simulink model "MPC_1_QuadrotorModel"  (R2023b)
settings: Solver=VariableStepAuto  StartTime=0.0  StopTime=60  FixedStep=0.0005  MaxStep=0.05  RelTol=1e-3
InitFcn:
  | nlobj = init_nmpc();
values from neighbouring files (symbols this model uses):
  A_flap = [c_a, c_b, 0 ... (first row only)    [LQR_calculate.m]    (also in LQR_feedback.m; LQR_linearized_test.m; MPC_test.m; MPC_test_1.m)
  A_ind = [c_d, 0, 0 ... (first row only)    [LQR_calculate.m]    (also in LQR_feedback.m; LQR_linearized_test.m; MPC_test.m; MPC_test_1.m)
  C_drag = 0    [LQR_calculate.m]    (also in LQR_feedback.m = C_drag_arr(i); LQR_linearized_test.m = C_drag_arr(i); MPC_test.m = C_drag_arr(i); MPC_test_1.m = C_drag_arr(i))
  demp = 0    [LQR_feedback.m]    (also in LQR_linearized_test.m; MPC_params.m; MPC_test_1.m; initQuadrotorData.m)
  forward_1 = 20    [LQR_feedback.m]    (also in LQR_linearized_test.m; MPC_test_1.m)
  forward_2 = 20    [LQR_feedback.m]    (also in LQR_linearized_test.m; MPC_test_1.m)
  g = 9.81    [LQR_calculate.m]    (also in LQR_feedback.m = 9.8; LQR_linearized_test.m = 9.8; LQR_testing_gpt.m; MPC_params.m = 9.8)
  Ix = m/3*a^2/12+2*0.045*l^2    (= 0.00211347222222)    [LQR_calculate.m]    (also in LQR_feedback.m; LQR_linearized_test.m; LQR_testing_gpt.m = 0.0081; MPC_params.m)
  Iy = m/3*a^2/12+4*0.045*l^2    (= 0.00413847222222)    [LQR_calculate.m]    (also in LQR_feedback.m = 0.00211347222222; LQR_linearized_test.m = 0.00211347222222; LQR_testing_gpt.m = 0.0081; MPC_params.m = 0.00211347222222)
  Iz = m/3*a^2/4+2*0.045*l^2    (= 0.00229041666667)    [LQR_calculate.m]    (also in LQR_feedback.m = 0.00431541666667; LQR_linearized_test.m = 0.00431541666667; LQR_testing_gpt.m = 0.0142; MPC_params.m = 0.00431541666667)
  J = 2.5*10^(-6)    (= 2.5e-06)    [LQR_calculate.m]    (also in LQR_feedback.m; LQR_linearized_test.m; MPC_params.m; MPC_test.m)
  Ke = ke    (= 0.0073)    [LQR_calculate.m]    (also in LQR_feedback.m = 0.00734; LQR_linearized_test.m = 0.00734; MPC_params.m = 0.00734; MPC_test.m)
  kf = ks*r^2*airDensity*Sblade/2    (= 1.57565625e-05)    [LQR_calculate.m]    (also in LQR_feedback.m; LQR_linearized_test.m; MPC_params.m; MPC_test.m)
  Km = kt    (= 0.0073)    [LQR_calculate.m]    (also in LQR_feedback.m = 0.00734; LQR_linearized_test.m = 0.00734; MPC_params.m = 0.00734; MPC_test.m)
  kv = 1300    [LQR_feedback.m]    (also in LQR_linearized_test.m; MPC_test_1.m; initQuadrotorData.m)
  L = La    (= 5e-05)    [LQR_calculate.m]    (also in LQR_feedback.m = 0.0001; LQR_linearized_test.m = 0.0001; MPC_params.m = 0.0001; MPC_test.m)
  l = 0.15    [LQR_calculate.m]    (also in LQR_feedback.m; LQR_linearized_test.m; MPC_params.m; MPC_test.m)
  m = size(B, 2)    [LQR_calculate.m]    (also in LQR_feedback.m = 0.65; LQR_linearized_test.m = 0.65; LQR_testing_gpt.m = 1; MPC_params.m = 0.65)
  maxU = 16    [LQR_calculate.m]    (also in LQR_feedback.m; LQR_linearized_test.m; MPC_params.m; MPC_test.m = 11)
  Mode = 3    [LQR_feedback.m]    (also in LQR_linearized_test.m; MPC_test_1.m = 1)
  N = params.N    [MPC_test_1.m]    (also in initQuadrotorData.m)
  phi0 = 0    [LQR_feedback.m]    (also in LQR_linearized_test.m; MPC_test_1.m)
  psi0 = pi/2    (= 1.57079632679)    [LQR_feedback.m]    (also in LQR_linearized_test.m; MPC_test_1.m = 0)
  Qc = diag([500, 500, 500, 1, 1, 1, 1, 1, 10, 1, 1, 1])    [MPC_test_1.m]
  R = eye(4)    [LQR_calculate.m]    (also in LQR_feedback.m = 0.058; LQR_linearized_test.m = 0.058; LQR_testing_gpt.m = diag([0.1, 10, 100, 10]); MPC_params.m = 0.058)
  Rc = diag([1, 1, 1, 1])    [LQR_feedback.m]    (also in LQR_linearized_test.m; MPC_test_1.m = diag([0.1, 0.1, 0.1, 0.1]))
  rho = 1.225    [LQR_calculate.m]    (also in LQR_feedback.m; LQR_linearized_test.m; MPC_params.m; MPC_test.m)
  S = l*c*4+a*b    (= 0.0169)    [LQR_calculate.m]    (also in LQR_feedback.m; LQR_linearized_test.m; MPC_params.m; MPC_test.m)
  theta0 = 0    [LQR_feedback.m]    (also in LQR_linearized_test.m; MPC_test_1.m)
  total_time = 60    [LQR_feedback.m]    (also in LQR_linearized_test.m; MPC_test_1.m)
  U_ref = repmat(u_nominal', params.N, 1)    [MPC_test_1.m]    (also in initQuadrotorData.m)
  up_down = 5    [LQR_feedback.m]    (also in LQR_linearized_test.m; MPC_test_1.m)
  x0 = 0    [LQR_feedback.m]    (also in LQR_linearized_test.m; MPC_test_1.m; init_nmpc.m = zeros(nx,1))
  y0 = 0    [LQR_feedback.m]    (also in LQR_linearized_test.m; MPC_test_1.m)
  z0 = 0    [LQR_feedback.m]    (also in LQR_linearized_test.m; MPC_test_1.m)
libraries: mpclib x1, sharedtransform x1
settings Model: Creator=Degra  LastModifiedBy=Degra

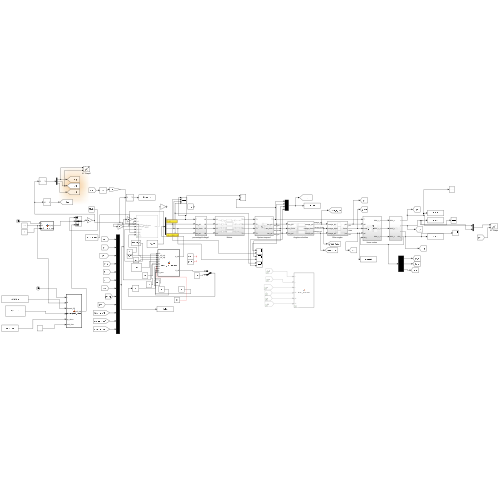
[thumbnail: Simulink's stored preview of the top-level diagram]
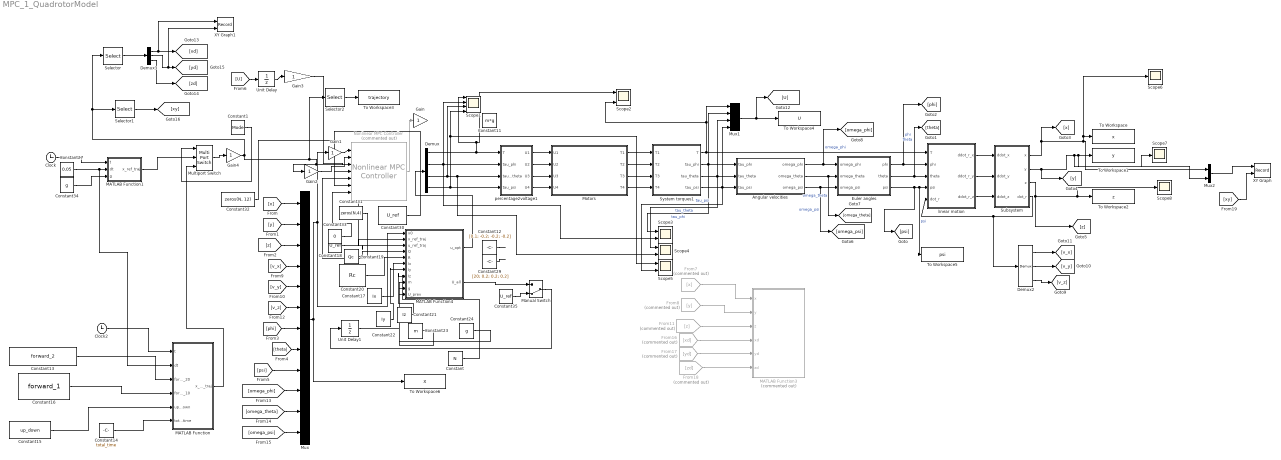
== system MPC_1_QuadrotorModel ==
  Angular velocities : Subsystem
  Clock : Clock
  Clock2 : Clock
  Constant : Constant  Value=N
  Constant1 : Constant  Value=Mode
  Constant11 : Constant  Value=m*g
  Constant12 : Constant  Value=[0.1; -0.2; -0.2; -0.2]
  Constant13 : Constant  Value=forward_2
  Constant14 : Constant  Value=total_time
  Constant15 : Constant  Value=up_down
  Constant16 : Constant  Value=forward_1
  Constant17 : Constant  Value=Ix
  Constant18 : Constant  Value=U_ref
  Constant19 : Constant  Value=Qc
  Constant20 : Constant  Value=Rc
  Constant21 : Constant  Value=Iz
  Constant22 : Constant  Value=Iy
  Constant23 : Constant  Value=m
  Constant24 : Constant  Value=g
  Constant27 : Constant  Value=0.05
  Constant29 : Constant  Value=[20; 0.2; 0.2; 0.2]
  Constant30 : Constant  Value=U_ref
  Constant31 : Constant  Value=zeros(N,4)
  Constant32 : Constant  Value=zeros(N, 12)
  Constant33 : Constant  Value=0
  Constant34 : Constant  Value=g
  Constant35 : Constant  Value=U_ref
  Demux : Demux
  Demux2 : Demux  Outputs=3
  Demux3 : Demux  Outputs=3
  Euler angles : Subsystem
  From11 : From  Commented=on  GotoTag=z
  From16 : From  Commented=on  GotoTag=xd
  From17 : From  Commented=on  GotoTag=yd
  From18 : From  Commented=on  GotoTag=zd
  From7 : From  Commented=on  GotoTag=x
  From8 : From  Commented=on  GotoTag=y
  Gain{,1..4} (5 alike) : Gain
  MATLAB Function : MATLAB Function  TreatAsAtomicUnit=on
  MATLAB Function1 : MATLAB Function  TreatAsAtomicUnit=on
  MATLAB Function3 : MATLAB Function  Commented=on  TreatAsAtomicUnit=on
  MATLAB Function4 : MATLAB Function  TreatAsAtomicUnit=on
  Manual Switch : ManualSwitch  CurrentSetting=0
  Motors : Subsystem
  Multiport Switch : MultiPortSwitch  Inputs=2  SaturateOnIntegerOverflow=off  InputSameDT=off
  Mux : Mux  Inputs=12
  Mux1 : Mux
  Mux2 : Mux  Inputs=2
  Nonlinear MPC Controller : mpclib/Nonlinear MPC Controller  Commented=on  nlmpcobj=nlobj  UseObjectTs=off  TsControl=0.01  UseMEX=off  md_enabled=off  mvtarget_enabled=on  param_enabled=off  cost_enabled=off  mvseq_enabled=off  stateseq_enabled=off  ovseq_enabled=off  slack_enabled=off  status_enabled=off  ov_min=off  ov_max=off  mv_min=off  mv_max=off  mvrate_min=off  mvrate_max=off  state_min=off  state_max=off  ov_weight=off  mv_weight=off  mvrate_weight=off  ecr_weight=off  nlp_initialize=on
  Scope1 : Scope  NumInputPorts=4
  Scope2 : Scope  NumInputPorts=3
  Scope3 : Scope  NumInputPorts=2
  Scope4 : Scope  NumInputPorts=2
  Scope5 : Scope  NumInputPorts=2
  Scope6 : Scope
  Scope7 : Scope
  Scope8 : Scope
  Selector : Selector  NumberOfDimensions=2  InputPortWidth=10  IndexOptions=Index vector (dialog),Index vector (dialog)  Indices=1,[1 2 3]  OutputSizes=1,1
  Selector1 : Selector  NumberOfDimensions=2  InputPortWidth=10  IndexOptions=Index vector (dialog),Index vector (dialog)  Indices=1,[1 2]  OutputSizes=1,1
  Selector2 : Selector  NumberOfDimensions=2  InputPortWidth=10  IndexOptions=Index vector (dialog),Select all  Indices=1,[1 2 3]  OutputSizes=1,1
  Subsystem : Subsystem
  System torques1 : Subsystem
  To Workspace : ToWorkspace  VariableName=x  SaveFormat=Timeseries  SampleTime=-1
  To Workspace1 : ToWorkspace  VariableName=y  SaveFormat=Timeseries  SampleTime=-1
  To Workspace2 : ToWorkspace  VariableName=z  SaveFormat=Timeseries  SampleTime=-1
  To Workspace3 : ToWorkspace  VariableName=trajectory  SaveFormat=Timeseries  SampleTime=-1
  To Workspace4 : ToWorkspace  VariableName=U  SaveFormat=Timeseries  SampleTime=-1
  To Workspace5 : ToWorkspace  VariableName=psi  SaveFormat=Timeseries  SampleTime=-1
  To Workspace6 : ToWorkspace  VariableName=X  SaveFormat=Timeseries  SampleTime=-1
  Unit Delay : UnitDelay  SampleTime=0.005  HasFrameUpgradeWarning=on
  Unit Delay1 : UnitDelay  InitialCondition=U_ref  SampleTime=-1  HasFrameUpgradeWarning=on
  XY Graph : Record  FileSettingsInternal="{\"entries\":[{\"content\":{\"excelSettings\":{\"content\":{},\"type\":\"Streamout.ExcelSettings\"}},\"type\":\"Streamout.FileSettingStorage\",\"uuid\":\"\"}],\"packageUris\":[\"http:\\/\\/schema.mathworks.com\\/mf0\\/streamout_blocks\\/R2020a\"],\"version\":\"1.0\"}"  Layout=[1 1]  SignalsInternal="{\"entries\":[{\"content\":{\"signals\":[{\"content\":{\"blockPath\":[],\"dimensions\":[2],\"domain\":\"\",\"hasChildren\":true,\"lineColor\":\"#ff6929\",\"port\":1,\"sid\":[\"\"],\"signalID\":267043,\"signalName\":\"Mux2\"},\"type\":\"RecordBlkView.Signal\",\"uuid\":\"\"},{\"content\":{\"blockPath\":[],\"channel\":[1],\"dimensions\":[2],\"domain\":\"\",\"lineColor\":\"#4dbeee\",\"parentID\":267043,\"plots\":[1],\"port\":1,\"sid\":[\"\"],\"signalID\":267044,\"signalName\":\"Mux2\"},\"type\":\"RecordBlkView.Signal\",\"uuid\":\"\"},{\"content\":{\"blockPath\":[],\"dimensions\":[1,2],\"domain\":\"\",\"hasChildren\":true,\"lineColor\":\"#64d413\",\"port\":2,\"sid\":[\"\"],\"signalID\":267048,\"signalName\":\"From19\"},\"type\":\"RecordBlkView.Signal\",\"uuid\":\"\"},{\"content\":{\"blockPath\":[],\"channel\":[1,1],\"dimensions\":[1,2],\"domain\":\"\",\"lineColor\":\"#fe330a\",\"parentID\":267048,\"plots\":[1],\"port\":2,\"sid\":[\"\"],\"signalID\":267049,\"signalName\":\"From19\"},\"type\":\"RecordBlkView.Signal\",\"uuid\":\"\"},{\"content\":{\"blockPath\":[],\"channel\":[2],\"dimensions\":[2],\"domain\":\"\",\"lineColor\":\"#77ac30\",\"parentID\":267043,\"plots\":[1],\"port\":1,\"sid\":[\"\"],\"signalID\":267099,\"signalName\":\"Mux2\"},\"type\":\"RecordBlkView.Signal\",\"uuid\":\"\"},{\"content\":{\"blockPath\":[],\"channel\":[1,2],\"dimensions\":[1,2],\"domain\":\"\",\"lineColor\":\"#a2142f\",\"parentID\":267048,\"plots\":[1],\"port\":2,\"sid\":[\"\"],\"signalID\":267100,\"signalName\":\"From19\"},\"type\":\"RecordBlkView.Signal\",\"uuid\":\"\"}]},\"type\":\"RecordBlkView.InputSignals\",\"uuid\":\"\"}],\"packageUris\":[\"http:\\/\\/schema.mathworks.com\\/mf0\\/streamout_blocks\\/R2020a\"],\"version\":\"1.0\"}"  VisualizationBindings="{\"xyplotplugin\":{\"info\":[{\"series\":[{\"bindingParametersList\":[{\"parameter\":\"X-Axis\",\"signalID\":267044,\"signalName\":\"Mux2(1)\"},{\"parameter\":\"Y-Axis\",\"signalID\":267099,\"signalName\":\"Mux2(2)\"}],\"seriesID\":23159},{\"bindingParametersList\":[{\"parameter\":\"X-Axis\",\"signalID\":267049,\"signalName\":\"From19(1,1)\"},{\"parameter\":\"Y-Axis\",\"signalID\":267100,\"signalName\":\"From19(1,2)\"}],\"seriesID\":40208}],\"subplotID\":1}]}}"  CompatibilityTag=XY
  XY Graph1 : Record  FileSettingsInternal="{\"entries\":[{\"content\":{\"excelSettings\":{\"content\":{},\"type\":\"Streamout.ExcelSettings\"}},\"type\":\"Streamout.FileSettingStorage\",\"uuid\":\"\"}],\"packageUris\":[\"http:\\/\\/schema.mathworks.com\\/mf0\\/streamout_blocks\\/R2020a\"],\"version\":\"1.0\"}"  Layout=[1 1]  SignalsInternal="{\"entries\":[{\"content\":{\"signals\":[{\"content\":{\"blockPath\":[],\"dimensions\":[1,1],\"domain\":\"\",\"lineColor\":\"#a2142f\",\"plots\":[1],\"port\":1,\"sid\":[\"\"],\"signalID\":267053,\"signalName\":\"Demux3:1\"},\"type\":\"RecordBlkView.Signal\",\"uuid\":\"\"},{\"content\":{\"blockPath\":[],\"dimensions\":[1,1],\"domain\":\"\",\"lineColor\":\"#139fff\",\"plots\":[1],\"port\":2,\"sid\":[\"\"],\"signalID\":267057,\"signalName\":\"Demux3:2\"},\"type\":\"RecordBlkView.Signal\",\"uuid\":\"\"}]},\"type\":\"RecordBlkView.InputSignals\",\"uuid\":\"\"}],\"packageUris\":[\"http:\\/\\/schema.mathworks.com\\/mf0\\/streamout_blocks\\/R2020a\"],\"version\":\"1.0\"}"  VisualizationBindings="{\"xyplotplugin\":{\"info\":[{\"series\":[{\"bindingParametersList\":[{\"parameter\":\"X-Axis\",\"signalID\":267053,\"signalName\":\"Demux3:1\"},{\"parameter\":\"Y-Axis\",\"signalID\":267057,\"signalName\":\"Demux3:2\"}],\"seriesID\":26950}],\"subplotID\":1}]}}"  CompatibilityTag=XY
  linear motion : Subsystem
  percentage2voltage1 : Subsystem
  wires:
  Angular velocities/1(omega_phi) -> [omega_phi], Euler angles/1(omega_phi)  "omega_phi"
  Angular velocities/2(omega_theta) -> [omega_theta], Euler angles/2(omega_theta)  "omega_theta"
  Angular velocities/3(omega_psi) -> [omega_psi], Euler angles/3(omega_psi)  "omega_psi"
  Euler angles/1(phi) -> [phi], linear motion/2(phi)  "phi"
  Euler angles/2(theta) -> [theta], linear motion/3(theta)  "theta"
  Euler angles/3(psi) -> [psi], To Workspace5/1, linear motion/4(psi)  "psi"
  linear motion/1(ddot_r_x) -> Subsystem/1(ddot_x)
  linear motion/2(ddot_r_y) -> Subsystem/2(ddot_y)
  linear motion/3(ddot_r_z) -> Subsystem/3(ddot_z)
  Subsystem/2(y) -> [y], Mux2/2, Scope7/1, To Workspace1/1
  Subsystem/3(z) -> [z], Scope8/1, To Workspace2/1
  Clock/1 -> MATLAB Function1/1(t)
  [x] -> Mux/1
  [z] -> Mux/3
  [y] -> Mux/2
  Mux/1 -> To Workspace6/1, MATLAB Function4/1(x0), Gain1/1
  [phi] -> Mux/7
  [theta] -> Mux/8
  [psi] -> Mux/9
  [omega_theta] -> Mux/11
  [omega_phi] -> Mux/10
  [omega_psi] -> Mux/12
  [v_z] -> Mux/6
  [v_y] -> Mux/5
  [v_x] -> Mux/4
  Constant1/1 -> Multiport Switch/1
  Demux/2 -> Scope3/2, percentage2voltage1/2(tau_phi), Scope1/2
  Demux/3 -> Scope4/2, percentage2voltage1/3(tau_theta), Scope1/3
  Demux/4 -> Scope5/1, Scope1/4, percentage2voltage1/4(tau_psi)
  Constant13/1 -> MATLAB Function/3(forward_20)
  Constant16/1 -> MATLAB Function/4(forward_10)
  Constant15/1 -> MATLAB Function/5(up_down)
  Constant14/1 -> MATLAB Function/6(total_time)
  Clock2/1 -> MATLAB Function/1(t)
  Subsystem/4(dot_r) -> Demux2/1, linear motion/5(dot_r)
  Demux2/3 -> [v_z]
  Demux2/2 -> [v_y]
  Demux2/1 -> [v_x]
  System torques1/4(tau_psi) -> Mux1/4, Scope5/2, Angular velocities/3(tau_psi)  "tau_psi"
  System torques1/3(tau_theta) -> Scope4/1, Mux1/3, Angular velocities/2(tau_theta)  "tau_theta"
  System torques1/2(tau_phi) -> Mux1/2, Scope3/1, Angular velocities/1(tau_phi)  "tau_phi"
  System torques1/1(T) -> Mux1/1, Scope2/3, linear motion/1(T)
  Motors/1(T1) -> System torques1/1(T1)
  Motors/2(T2) -> System torques1/2(T2)
  Motors/3(T3) -> System torques1/3(T3)
  Motors/4(T4) -> System torques1/4(T4)
  percentage2voltage1/2(U2) -> Motors/2(U2)
  percentage2voltage1/3(U3) -> Motors/3(U3)
  percentage2voltage1/4(U4) -> Motors/4(U4)
  Mux1/1 -> [U], To Workspace4/1
  Constant18/1 -> MATLAB Function4/3(u_ref_traj)
  Constant19/1 -> MATLAB Function4/4(Q)
  Constant20/1 -> MATLAB Function4/5(R)
  Constant17/1 -> MATLAB Function4/6(Ix)
  Constant22/1 -> MATLAB Function4/7(Iy)
  Constant21/1 -> MATLAB Function4/8(Iz)
  Constant23/1 -> MATLAB Function4/9(m)
  Constant24/1 -> MATLAB Function4/10(g)
  Constant/1 -> ?
  Constant27/1 -> MATLAB Function/2(dt), MATLAB Function1/2(dt)
  percentage2voltage1/1(U1) -> Motors/1(U1)
  Demux/1 -> percentage2voltage1/1(T), Scope2/1, Scope1/1
  Constant12/1 -> ?
  Constant29/1 -> ?
  Nonlinear MPC Controller/1 -> Gain/1
  Gain1/1 -> Nonlinear MPC Controller/1
  Gain2/1 -> Nonlinear MPC Controller/2
  Constant30/1 -> Nonlinear MPC Controller/4
  Constant31/1 -> Nonlinear MPC Controller/5
  Constant32/1 -> Nonlinear MPC Controller/6
  Constant33/1 -> Nonlinear MPC Controller/7
  Gain3/1 -> Nonlinear MPC Controller/3
  Unit Delay/1 -> Gain3/1
  [U] -> Unit Delay/1
  MATLAB Function4/1(u_opt) -> Demux/1
  From7/1 -> MATLAB Function3/1(x)
  From8/1 -> MATLAB Function3/2(y)
  From11/1 -> MATLAB Function3/3(z)
  From16/1 -> MATLAB Function3/4(xd)
  From17/1 -> MATLAB Function3/5(yd)
  From18/1 -> MATLAB Function3/6(zd)
  Demux3/1 -> XY Graph1/1, [xd]
  Demux3/2 -> XY Graph1/2, [yd]
  Demux3/3 -> [zd]
  Selector/1 -> Demux3/1
  Selector1/1 -> [xy]
  Subsystem/1(x) -> [x], Mux2/1, Scope6/1, To Workspace/1
  Mux2/1 -> XY Graph/1
  [xy] -> XY Graph/2
  Constant34/1 -> MATLAB Function1/3(g)
  Unit Delay1/1 -> MATLAB Function4/11(U_prev)
  Manual Switch/1 -> Unit Delay1/1
  MATLAB Function4/2(U_all) -> Manual Switch/1
  Constant35/1 -> Manual Switch/2
  Gain4/1 -> Selector2/1, Gain2/1, MATLAB Function4/2(x_ref_traj), Selector1/1, Selector/1
  Multiport Switch/1 -> Gain4/1
  MATLAB Function1/1(x_ref_traj) -> Multiport Switch/2
  MATLAB Function/1(x_ref_traj) -> Multiport Switch/3
  Selector2/1 -> To Workspace3/1

== system MPC_1_QuadrotorModel/Angular velocities ==
  tau_phi : Inport
  tau_theta : Inport  Port=2
  tau_psi : Inport  Port=3
  Subsystem1 : Subsystem
  Subsystem2 : Subsystem
  Subsystem3 : Subsystem
  omega_phi : Outport
  omega_theta : Outport  Port=2
  omega_psi : Outport  Port=3
  wires:
  Subsystem2/1(omega_theta) -> omega_theta/1, Subsystem1/2(omega_theta), Subsystem3/3(omega_theta)  "omega_theta"
  tau_theta/1 -> Subsystem2/1(tau_theta)
  Subsystem1/1(omega_phi) -> omega_phi/1, Subsystem3/2(omega_phi), Subsystem2/2(omega_phi)  "omega_phi"
  Subsystem3/1(omega_psi) -> omega_psi/1, Subsystem2/3(omega_psi), Subsystem1/3(omega_psi)  "omega_psi"
  tau_phi/1 -> Subsystem1/1(tau_phi)
  tau_psi/1 -> Subsystem3/1(tau_psi)

== system MPC_1_QuadrotorModel/Euler angles ==
  omega_phi : Inport
  omega_theta : Inport  Port=2
  omega_psi : Inport  Port=3
  Subsystem1 : Subsystem
  Subsystem2 : Subsystem
  Subsystem3 : Subsystem
  phi : Outport
  theta : Outport  Port=2
  psi : Outport  Port=3
  wires:
  Subsystem2/1(theta) -> theta/1, Subsystem1/2(theta), Subsystem3/4(theta)  "theta"
  Subsystem1/1(phi) -> phi/1, Subsystem3/1(phi), Subsystem2/1(phi)  "phi"
  omega_theta/1 -> Subsystem3/2(omega_theta), Subsystem1/3(omega_theta), Subsystem2/2(omega_theta)
  omega_psi/1 -> Subsystem2/3(omega_psi), Subsystem3/3(omega_psi), Subsystem1/4(omega_psi)
  omega_phi/1 -> Subsystem1/1(omega_phi)
  Subsystem3/1(psi) -> psi/1  "psi"

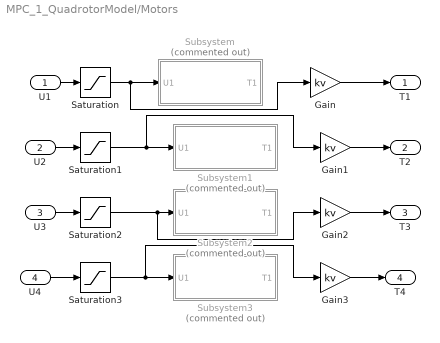
== system MPC_1_QuadrotorModel/Motors ==
  U1 : Inport
  U2 : Inport  Port=2
  U3 : Inport  Port=3
  U4 : Inport  Port=4
  Gain{,1..3} (4 alike) : Gain  Gain=kv
  Saturation{,1..3} (4 alike) : Saturate  UpperLimit=maxU  LowerLimit=-maxU
  Subsystem : Subsystem  Commented=on
  Subsystem1 : Subsystem  Commented=on
  Subsystem2 : Subsystem  Commented=on
  Subsystem3 : Subsystem  Commented=on
  T1 : Outport
  T2 : Outport  Port=2
  T3 : Outport  Port=3
  T4 : Outport  Port=4
  wires:
  U4/1 -> Saturation3/1
  U1/1 -> Saturation/1
  U3/1 -> Saturation2/1
  U2/1 -> Saturation1/1
  Gain/1 -> T1/1
  Gain1/1 -> T2/1
  Gain2/1 -> T3/1
  Gain3/1 -> T4/1
  Saturation/1 -> Gain/1, Subsystem/1(U1)
  Saturation1/1 -> Gain1/1, Subsystem1/1(U1)
  Saturation2/1 -> Gain2/1, Subsystem2/1(U1)
  Saturation3/1 -> Gain3/1, Subsystem3/1(U1)

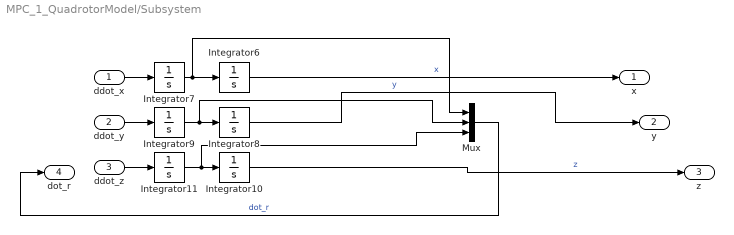
== system MPC_1_QuadrotorModel/Subsystem ==
  ddot_x : Inport
  ddot_y : Inport  Port=2
  ddot_z : Inport  Port=3
  Integrator10 : Integrator  InitialCondition=z0
  Integrator11 : Integrator
  Integrator6 : Integrator  InitialCondition=x0
  Integrator7 : Integrator
  Integrator8 : Integrator  InitialCondition=y0
  Integrator9 : Integrator
  Mux : Mux  Inputs=3
  x : Outport
  y : Outport  Port=2
  z : Outport  Port=3
  dot_r : Outport  Port=4
  wires:
  Integrator9/1 -> Mux/2, Integrator8/1
  Integrator7/1 -> Mux/1, Integrator6/1
  Integrator10/1 -> z/1  "z"
  Integrator11/1 -> Mux/3, Integrator10/1
  Integrator8/1 -> y/1  "y"
  ddot_x/1 -> Integrator7/1
  Mux/1 -> dot_r/1  "dot_r"
  Integrator6/1 -> x/1  "x"
  ddot_y/1 -> Integrator9/1
  ddot_z/1 -> Integrator11/1

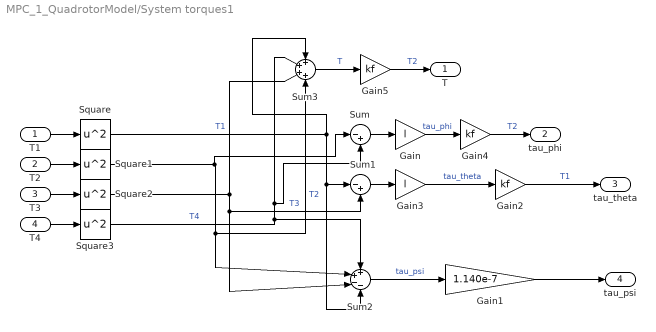
== system MPC_1_QuadrotorModel/System torques1 ==
  T1 : Inport
  T2 : Inport  Port=2
  T3 : Inport  Port=3
  T4 : Inport  Port=4
  Gain : Gain  Gain=l
  Gain1 : Gain  Gain=1.140e-7
  Gain2 : Gain  Gain=kf
  Gain3 : Gain  Gain=l
  Gain4 : Gain  Gain=kf
  Gain5 : Gain  Gain=kf
  Square{,1..3} (4 alike) : Math  Operator=square
  Sum : Sum  Inputs=|-+
  Sum1 : Sum  Inputs=|-+
  Sum2 : Sum  Inputs=++--
  Sum3 : Sum  Inputs=++++
  T : Outport
  tau_phi : Outport  Port=2
  tau_theta : Outport  Port=3
  tau_psi : Outport  Port=4
  wires:
  T3/1 -> Square2/1
  T4/1 -> Square3/1
  Sum2/1 -> Gain1/1  "tau_psi"
  T1/1 -> Square/1
  Sum/1 -> Gain/1
  Sum1/1 -> Gain3/1
  Sum3/1 -> Gain5/1  "T"
  T2/1 -> Square1/1
  Gain3/1 -> Gain2/1  "tau_theta"
  Gain/1 -> Gain4/1  "tau_phi"
  Gain1/1 -> tau_psi/1
  Square/1 -> Sum1/1, Sum2/4, Sum3/1  "T1"
  Square1/1 -> Sum/1, Sum2/2, Sum3/4  "T2"
  Square2/1 -> Sum1/2, Sum2/3, Sum3/3  "T3"
  Square3/1 -> Sum/2, Sum3/2, Sum2/1  "T4"
  Gain4/1 -> tau_phi/1  "T2"
  Gain2/1 -> tau_theta/1  "T1"
  Gain5/1 -> T/1  "T2"

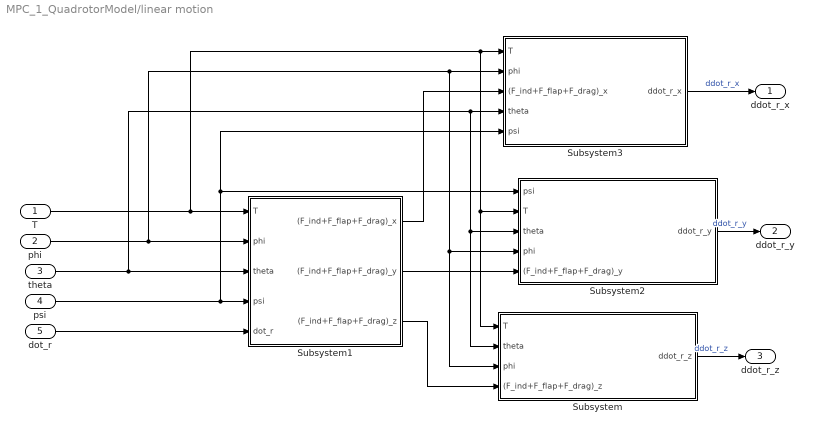
== system MPC_1_QuadrotorModel/linear motion ==
  T : Inport
  phi : Inport  Port=2
  theta : Inport  Port=3
  psi : Inport  Port=4
  dot_r : Inport  Port=5
  Subsystem : Subsystem
  Subsystem1 : Subsystem
  Subsystem2 : Subsystem
  Subsystem3 : Subsystem
  ddot_r_x : Outport
  ddot_r_y : Outport  Port=2
  ddot_r_z : Outport  Port=3
  wires:
  T/1 -> Subsystem/1(T), Subsystem2/2(T), Subsystem3/1(T), Subsystem1/1(T)
  theta/1 -> Subsystem/2(theta), Subsystem2/3(theta), Subsystem3/4(theta), Subsystem1/3(theta)
  phi/1 -> Subsystem/3(phi), Subsystem2/4(phi), Subsystem3/2(phi), Subsystem1/2(phi)
  Subsystem1/3((F_ind+F_flap+F_drag)_z) -> Subsystem/4((F_ind+F_flap+F_drag)_z)
  psi/1 -> Subsystem3/5(psi), Subsystem2/1(psi), Subsystem1/4(psi)
  dot_r/1 -> Subsystem1/5(dot_r)
  Subsystem1/2((F_ind+F_flap+F_drag)_y) -> Subsystem2/5((F_ind+F_flap+F_drag)_y)
  Subsystem1/1((F_ind+F_flap+F_drag)_x) -> Subsystem3/3((F_ind+F_flap+F_drag)_x)
  Subsystem3/1(ddot_r_x) -> ddot_r_x/1  "ddot_r_x"
  Subsystem2/1(ddot_r_y) -> ddot_r_y/1  "ddot_r_y"
  Subsystem/1(ddot_r_z) -> ddot_r_z/1  "ddot_r_z"

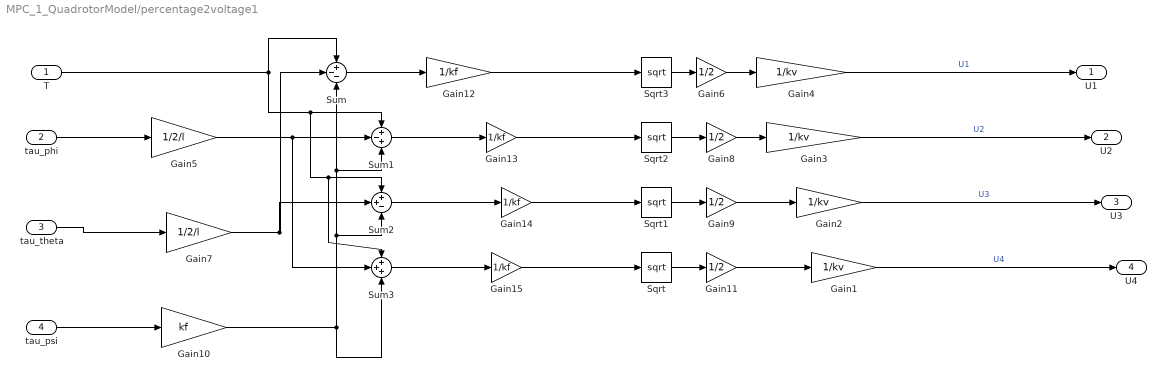
== system MPC_1_QuadrotorModel/percentage2voltage1 ==
  T : Inport
  tau_phi : Inport  Port=2
  tau_theta : Inport  Port=3
  tau_psi : Inport  Port=4
  Gain{1..4} (4 alike) : Gain  Gain=1/kv
  Gain10 : Gain  Gain=kf
  Gain{6,8..9,11} (4 alike) : Gain  Gain=1/2
  Gain{12..15} (4 alike) : Gain  Gain=1/kf
  Gain5 : Gain  Gain=1/2/l
  Gain7 : Gain  Gain=1/2/l
  Sqrt{,1..3} (4 alike) : Sqrt
  Sum : Sum  Inputs=+--
  Sum1 : Sum  Inputs=+-+
  Sum2 : Sum  Inputs=++-
  Sum3 : Sum  Inputs=+++
  U1 : Outport
  U2 : Outport  Port=2
  U3 : Outport  Port=3
  U4 : Outport  Port=4
  wires:
  Gain2/1 -> U3/1  "U3"
  Gain4/1 -> U1/1  "U1"
  Gain3/1 -> U2/1  "U2"
  Gain1/1 -> U4/1  "U4"
  Sum3/1 -> Gain15/1
  Sum2/1 -> Gain14/1
  tau_phi/1 -> Gain5/1
  tau_theta/1 -> Gain7/1
  tau_psi/1 -> Gain10/1
  Gain10/1 -> Sum3/3, Sum1/3, Sum/3, Sum2/3
  Sqrt/1 -> Gain11/1
  Sqrt1/1 -> Gain9/1
  Sqrt2/1 -> Gain8/1
  Sqrt3/1 -> Gain6/1
  Gain6/1 -> Gain4/1
  Gain8/1 -> Gain3/1
  Gain9/1 -> Gain2/1
  Gain11/1 -> Gain1/1
  Sum/1 -> Gain12/1
  Sum1/1 -> Gain13/1
  Gain14/1 -> Sqrt1/1
  Gain15/1 -> Sqrt/1
  Gain5/1 -> Sum3/2, Sum1/2
  Gain7/1 -> Sum2/2, Sum/2
  T/1 -> Sum3/1, Sum2/1, Sum1/1, Sum/1
  Gain12/1 -> Sqrt3/1
  Gain13/1 -> Sqrt2/1

== system MPC_1_QuadrotorModel/Angular velocities/Subsystem1 ==
  tau_phi : Inport
  omega_theta : Inport  Port=2
  omega_psi : Inport  Port=3
  Gain : Gain  Gain=Iy-Iz
  Gain1 : Gain  Gain=1/Ix
  Integrator12 : Integrator
  Product : Product
  Sum : Sum  Inputs=|++
  omega_phi : Outport
  wires:
  Gain/1 -> Sum/2
  omega_theta/1 -> Product/1
  Product/1 -> Gain/1
  Sum/1 -> Gain1/1  "dot_omega_phi"
  tau_phi/1 -> Sum/1
  omega_psi/1 -> Product/2
  Gain1/1 -> Integrator12/1
  Integrator12/1 -> omega_phi/1  "omega_phi"

== system MPC_1_QuadrotorModel/Angular velocities/Subsystem2 ==
  tau_theta : Inport
  omega_phi : Inport  Port=2
  omega_psi : Inport  Port=3
  Gain : Gain  Gain=Iz-Ix
  Gain1 : Gain  Gain=1/Iy
  Integrator12 : Integrator
  Product : Product
  Sum : Sum  Inputs=|++
  omega_theta : Outport
  wires:
  Gain/1 -> Sum/2
  Sum/1 -> Gain1/1  "omega_theta"
  omega_phi/1 -> Product/1
  Product/1 -> Gain/1
  tau_theta/1 -> Sum/1
  omega_psi/1 -> Product/2
  Gain1/1 -> Integrator12/1
  Integrator12/1 -> omega_theta/1  "omega_theta"

== system MPC_1_QuadrotorModel/Angular velocities/Subsystem3 ==
  tau_psi : Inport
  omega_phi : Inport  Port=2
  omega_theta : Inport  Port=3
  Gain : Gain  Gain=Ix-Iy
  Gain1 : Gain  Gain=1/Iz
  Integrator12 : Integrator
  Product : Product
  Sum : Sum  Inputs=|++
  omega_psi : Outport
  wires:
  Gain/1 -> Sum/2
  omega_phi/1 -> Product/1
  Product/1 -> Gain/1
  Sum/1 -> Gain1/1  "dot_omega_psi"
  tau_psi/1 -> Sum/1
  omega_theta/1 -> Product/2
  Gain1/1 -> Integrator12/1
  Integrator12/1 -> omega_psi/1  "omega_psi"

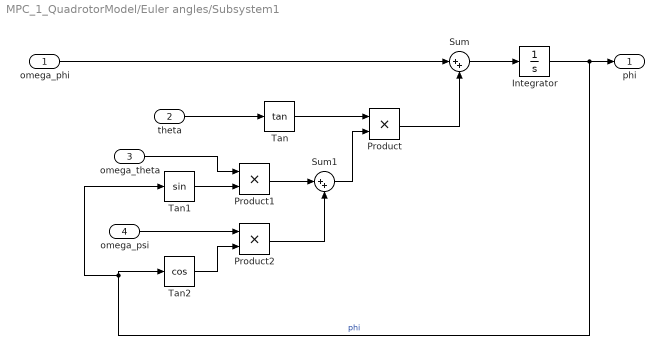
== system MPC_1_QuadrotorModel/Euler angles/Subsystem1 ==
  omega_phi : Inport
  theta : Inport  Port=2
  omega_theta : Inport  Port=3
  omega_psi : Inport  Port=4
  Integrator : Integrator  InitialCondition=phi0
  Product : Product
  Product1 : Product
  Product2 : Product
  Sum : Sum  Inputs=|++
  Sum1 : Sum  Inputs=|++
  Tan : Trigonometry  Operator=tan
  Tan1 : Trigonometry
  Tan2 : Trigonometry  Operator=cos
  phi : Outport
  wires:
  Product2/1 -> Sum1/2
  Tan1/1 -> Product1/2
  Sum/1 -> Integrator/1
  Sum1/1 -> Product/2
  Tan/1 -> Product/1
  Tan2/1 -> Product2/2
  Product1/1 -> Sum1/1
  omega_psi/1 -> Product2/1
  omega_theta/1 -> Product1/1
  Integrator/1 -> Tan1/1, Tan2/1, phi/1  "phi"
  theta/1 -> Tan/1
  omega_phi/1 -> Sum/1
  Product/1 -> Sum/2

== system MPC_1_QuadrotorModel/Euler angles/Subsystem2 ==
  phi : Inport
  omega_theta : Inport  Port=2
  omega_psi : Inport  Port=3
  Integrator : Integrator  InitialCondition=theta0
  Product1 : Product
  Product2 : Product
  Sum1 : Sum  Inputs=|+-
  Tan1 : Trigonometry  Operator=cos
  Tan2 : Trigonometry
  theta : Outport
  wires:
  Product2/1 -> Sum1/2
  Tan1/1 -> Product1/2
  Tan2/1 -> Product2/2
  Product1/1 -> Sum1/1
  omega_psi/1 -> Product2/1
  Integrator/1 -> theta/1  "theta"
  phi/1 -> Tan2/1, Tan1/1
  omega_theta/1 -> Product1/1
  Sum1/1 -> Integrator/1

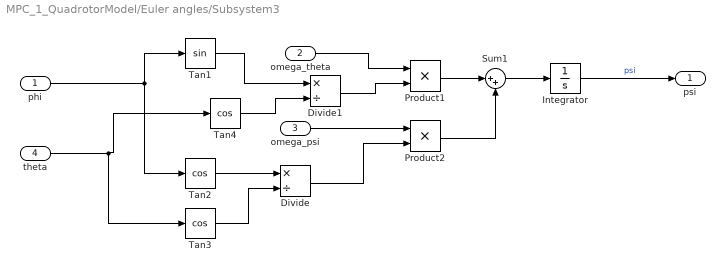
== system MPC_1_QuadrotorModel/Euler angles/Subsystem3 ==
  phi : Inport
  omega_theta : Inport  Port=2
  omega_psi : Inport  Port=3
  theta : Inport  Port=4
  Divide : Product  Inputs=*/
  Divide1 : Product  Inputs=*/
  Integrator : Integrator  InitialCondition=psi0
  Product1 : Product
  Product2 : Product
  Sum1 : Sum  Inputs=|++
  Tan1 : Trigonometry
  Tan2 : Trigonometry  Operator=cos
  Tan3 : Trigonometry  Operator=cos
  Tan4 : Trigonometry  Operator=cos
  psi : Outport
  wires:
  Product2/1 -> Sum1/2
  Product1/1 -> Sum1/1
  omega_psi/1 -> Product2/1
  Integrator/1 -> psi/1  "psi"
  phi/1 -> Tan1/1, Tan2/1
  theta/1 -> Tan4/1, Tan3/1
  Divide/1 -> Product2/2
  Tan2/1 -> Divide/1
  Tan3/1 -> Divide/2
  Divide1/1 -> Product1/2
  Tan1/1 -> Divide1/1
  Tan4/1 -> Divide1/2
  omega_theta/1 -> Product1/1
  Sum1/1 -> Integrator/1

== system MPC_1_QuadrotorModel/Motors/Subsystem ==
  U1 : Inport
  Add : Sum  Inputs=+--
  Add1 : Sum  Inputs=+-
  Gain : Gain  Gain=demp
  Gain1 : Gain  Gain=Km
  Gain2 : Gain  Gain=1/L
  Gain3 : Gain  Gain=Ke
  Gain5 : Gain  Gain=R
  Gain6 : Gain  Gain=1/J
  Integrator : Integrator
  Integrator1 : Integrator
  T1 : Outport
  wires:
  Gain2/1 -> Integrator/1
  Add/1 -> Gain2/1
  Integrator/1 -> Gain1/1, Gain5/1
  Gain5/1 -> Add/3
  U1/1 -> Add/1
  Gain1/1 -> Add1/1
  Add1/1 -> Gain6/1
  Integrator1/1 -> T1/1, Gain3/1, Gain/1
  Gain3/1 -> Add/2
  Gain/1 -> Add1/2
  Gain6/1 -> Integrator1/1

== system MPC_1_QuadrotorModel/Motors/Subsystem1 ==
  U1 : Inport
  Add : Sum  Inputs=+--
  Add1 : Sum  Inputs=+-
  Gain : Gain  Gain=demp
  Gain1 : Gain  Gain=Km
  Gain2 : Gain  Gain=1/L
  Gain3 : Gain  Gain=Ke
  Gain5 : Gain  Gain=R
  Gain6 : Gain  Gain=1/J
  Integrator : Integrator
  Integrator1 : Integrator
  T1 : Outport
  wires:
  Gain2/1 -> Integrator/1
  Add/1 -> Gain2/1
  Integrator/1 -> Gain1/1, Gain5/1
  Gain5/1 -> Add/3
  U1/1 -> Add/1
  Gain1/1 -> Add1/1
  Add1/1 -> Gain6/1
  Integrator1/1 -> T1/1, Gain3/1, Gain/1
  Gain3/1 -> Add/2
  Gain/1 -> Add1/2
  Gain6/1 -> Integrator1/1

== system MPC_1_QuadrotorModel/Motors/Subsystem2 ==
  U1 : Inport
  Add : Sum  Inputs=+--
  Add1 : Sum  Inputs=+-
  Gain : Gain  Gain=demp
  Gain1 : Gain  Gain=Km
  Gain2 : Gain  Gain=1/L
  Gain3 : Gain  Gain=Ke
  Gain5 : Gain  Gain=R
  Gain6 : Gain  Gain=1/J
  Integrator : Integrator
  Integrator1 : Integrator
  T1 : Outport
  wires:
  Gain2/1 -> Integrator/1
  Add/1 -> Gain2/1
  Integrator/1 -> Gain1/1, Gain5/1
  Gain5/1 -> Add/3
  U1/1 -> Add/1
  Gain1/1 -> Add1/1
  Add1/1 -> Gain6/1
  Integrator1/1 -> T1/1, Gain3/1, Gain/1
  Gain3/1 -> Add/2
  Gain/1 -> Add1/2
  Gain6/1 -> Integrator1/1

== system MPC_1_QuadrotorModel/Motors/Subsystem3 ==
  U1 : Inport
  Add : Sum  Inputs=+--
  Add1 : Sum  Inputs=+-
  Gain : Gain  Gain=demp
  Gain1 : Gain  Gain=Km
  Gain2 : Gain  Gain=1/L
  Gain3 : Gain  Gain=Ke
  Gain5 : Gain  Gain=R
  Gain6 : Gain  Gain=1/J
  Integrator : Integrator
  Integrator1 : Integrator
  T1 : Outport
  wires:
  Gain2/1 -> Integrator/1
  Add/1 -> Gain2/1
  Integrator/1 -> Gain1/1, Gain5/1
  Gain5/1 -> Add/3
  U1/1 -> Add/1
  Gain1/1 -> Add1/1
  Add1/1 -> Gain6/1
  Integrator1/1 -> T1/1, Gain3/1, Gain/1
  Gain3/1 -> Add/2
  Gain/1 -> Add1/2
  Gain6/1 -> Integrator1/1

== system MPC_1_QuadrotorModel/linear motion/Subsystem ==
  T : Inport
  theta : Inport  Port=2
  phi : Inport  Port=3
  (F_ind+F_flap+F_drag)_z : Inport  Port=4
  Constant4 : Constant  Value=m*g
  Cos4 : Trigonometry  Operator=cos
  Cos5 : Trigonometry  Operator=cos
  Gain4 : Gain  Gain=1/m
  Product2 : Product  Inputs=3
  Sum2 : Sum  Inputs=|+--
  ddot_r_z : Outport
  wires:
  Product2/1 -> Sum2/1
  phi/1 -> Cos4/1
  theta/1 -> Cos5/1
  T/1 -> Product2/1
  Cos4/1 -> Product2/2
  Constant4/1 -> Sum2/3
  Cos5/1 -> Product2/3
  (F_ind+F_flap+F_drag)_z/1 -> Sum2/2
  Sum2/1 -> Gain4/1
  Gain4/1 -> ddot_r_z/1  "ddot_r_z"

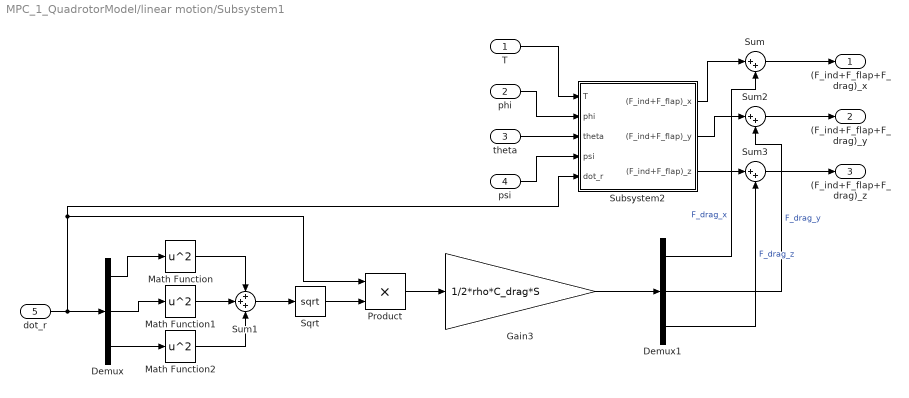
== system MPC_1_QuadrotorModel/linear motion/Subsystem1 ==
  T : Inport
  phi : Inport  Port=2
  theta : Inport  Port=3
  psi : Inport  Port=4
  dot_r : Inport  Port=5
  Demux : Demux  Outputs=3
  Demux1 : Demux  Outputs=3
  Gain3 : Gain  Gain=1/2*rho*C_drag*S
  Math Function : Math  Operator=square
  Math Function1 : Math  Operator=square
  Math Function2 : Math  Operator=square
  Product : Product
  Sqrt : Sqrt
  Subsystem2 : Subsystem
  Sum : Sum  Inputs=|++
  Sum1 : Sum  Inputs=+++
  Sum2 : Sum  Inputs=|++
  Sum3 : Sum  Inputs=|++
  (F_ind+F_flap+F_drag)_x : Outport
  (F_ind+F_flap+F_drag)_y : Outport  Port=2
  (F_ind+F_flap+F_drag)_z : Outport  Port=3
  wires:
  Demux1/2 -> Sum2/2  "F_drag_y"
  dot_r/1 -> Product/1, Subsystem2/5(dot_r), Demux/1
  Math Function1/1 -> Sum1/2
  Demux/1 -> Math Function/1
  Demux/2 -> Math Function1/1
  Sum1/1 -> Sqrt/1
  Math Function/1 -> Sum1/1
  Demux/3 -> Math Function2/1
  Demux1/3 -> Sum3/2  "F_drag_z"
  Subsystem2/2((F_ind+F_flap)_y) -> Sum2/1
  Math Function2/1 -> Sum1/3
  Sqrt/1 -> Product/2
  phi/1 -> Subsystem2/2(phi)
  Product/1 -> Gain3/1
  T/1 -> Subsystem2/1(T)
  theta/1 -> Subsystem2/3(theta)
  psi/1 -> Subsystem2/4(psi)
  Gain3/1 -> Demux1/1
  Subsystem2/1((F_ind+F_flap)_x) -> Sum/1
  Subsystem2/3((F_ind+F_flap)_z) -> Sum3/1
  Demux1/1 -> Sum/2  "F_drag_x"
  Sum/1 -> (F_ind+F_flap+F_drag)_x/1
  Sum2/1 -> (F_ind+F_flap+F_drag)_y/1
  Sum3/1 -> (F_ind+F_flap+F_drag)_z/1

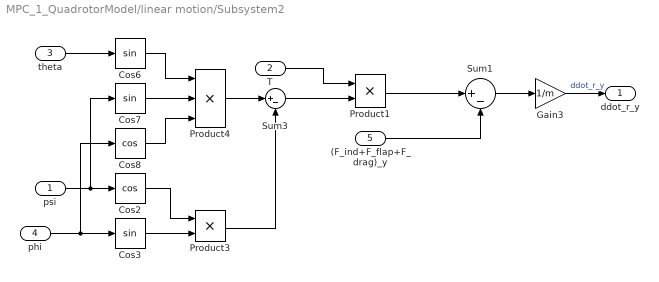
== system MPC_1_QuadrotorModel/linear motion/Subsystem2 ==
  psi : Inport
  T : Inport  Port=2
  theta : Inport  Port=3
  phi : Inport  Port=4
  (F_ind+F_flap+F_drag)_y : Inport  Port=5
  Cos2 : Trigonometry  Operator=cos
  Cos3 : Trigonometry
  Cos6 : Trigonometry
  Cos7 : Trigonometry
  Cos8 : Trigonometry  Operator=cos
  Gain3 : Gain  Gain=1/m
  Product1 : Product
  Product3 : Product
  Product4 : Product  Inputs=3
  Sum1 : Sum  Inputs=|+-
  Sum3 : Sum  Inputs=|+-
  ddot_r_y : Outport
  wires:
  Cos6/1 -> Product4/1
  theta/1 -> Cos6/1
  psi/1 -> Cos7/1, Cos2/1
  Cos7/1 -> Product4/2
  Sum1/1 -> Gain3/1
  phi/1 -> Cos8/1, Cos3/1
  Cos8/1 -> Product4/3
  Cos2/1 -> Product3/1
  Cos3/1 -> Product3/2
  Product4/1 -> Sum3/1
  Product3/1 -> Sum3/2
  T/1 -> Product1/1
  Sum3/1 -> Product1/2
  Product1/1 -> Sum1/1
  (F_ind+F_flap+F_drag)_y/1 -> Sum1/2
  Gain3/1 -> ddot_r_y/1  "ddot_r_y"

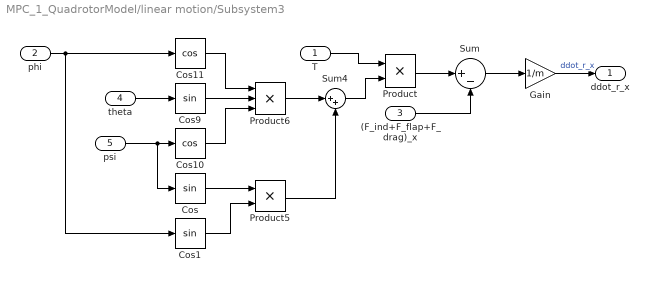
== system MPC_1_QuadrotorModel/linear motion/Subsystem3 ==
  T : Inport
  phi : Inport  Port=2
  (F_ind+F_flap+F_drag)_x : Inport  Port=3
  theta : Inport  Port=4
  psi : Inport  Port=5
  Cos : Trigonometry
  Cos1 : Trigonometry
  Cos10 : Trigonometry  Operator=cos
  Cos11 : Trigonometry  Operator=cos
  Cos9 : Trigonometry
  Gain : Gain  Gain=1/m
  Product : Product
  Product5 : Product
  Product6 : Product  Inputs=3
  Sum : Sum  Inputs=|+-
  Sum4 : Sum  Inputs=|++
  ddot_r_x : Outport
  wires:
  theta/1 -> Cos9/1
  Cos/1 -> Product5/1
  psi/1 -> Cos10/1, Cos/1
  Cos11/1 -> Product6/1
  Sum/1 -> Gain/1
  (F_ind+F_flap+F_drag)_x/1 -> Sum/2
  phi/1 -> Cos11/1, Cos1/1
  Cos1/1 -> Product5/2
  Cos9/1 -> Product6/2
  Cos10/1 -> Product6/3
  Product6/1 -> Sum4/1
  Product5/1 -> Sum4/2
  T/1 -> Product/1
  Sum4/1 -> Product/2
  Product/1 -> Sum/1
  Gain/1 -> ddot_r_x/1  "ddot_r_x"

== system MPC_1_QuadrotorModel/linear motion/Subsystem1/Subsystem2 ==
  T : Inport
  phi : Inport  Port=2
  theta : Inport  Port=3
  psi : Inport  Port=4
  dot_r : Inport  Port=5
  Demux : Demux  Outputs=3
  Subsystem1 : Subsystem
  (F_ind+F_flap)_x : Outport
  (F_ind+F_flap)_y : Outport  Port=2
  (F_ind+F_flap)_z : Outport  Port=3
  wires:
  T/1 -> Subsystem1/5(T)
  Subsystem1/1(F_ind+F_flap) -> Demux/1
  psi/1 -> Subsystem1/3(psi)
  Demux/2 -> (F_ind+F_flap)_y/1  "(F_ind+F_flap)_y"
  dot_r/1 -> Subsystem1/4(dot_r)
  theta/1 -> Subsystem1/2(theta)
  phi/1 -> Subsystem1/1(phi)
  Demux/1 -> (F_ind+F_flap)_x/1  "(F_ind+F_flap)_x"
  Demux/3 -> (F_ind+F_flap)_z/1  "(F_ind+F_flap)_z"

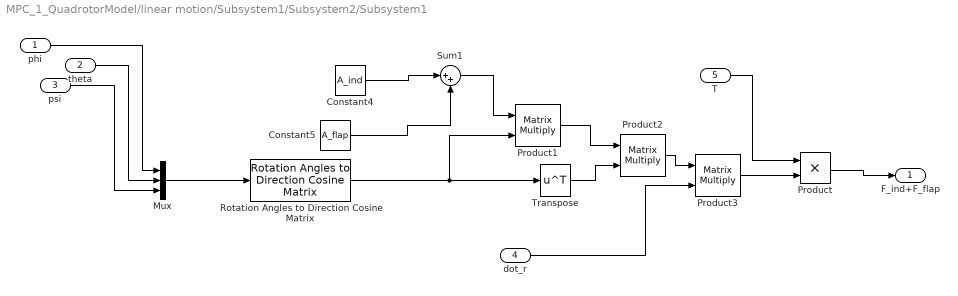
== system MPC_1_QuadrotorModel/linear motion/Subsystem1/Subsystem2/Subsystem1 ==
  phi : Inport
  theta : Inport  Port=2
  psi : Inport  Port=3
  dot_r : Inport  Port=4
  T : Inport  Port=5
  Constant4 : Constant  Value=A_ind
  Constant5 : Constant  Value=A_flap
  Mux : Mux  Inputs=3
  Product : Product
  Product1 : Product  Multiplication=Matrix(*)
  Product2 : Product  Multiplication=Matrix(*)
  Product3 : Product  Multiplication=Matrix(*)
  Rotation Angles to Direction Cosine Matrix : sharedtransform/Rotation Angles to Direction Cosine Matrix  rotationOrder=ZYX  aMode=aMode
  Sum1 : Sum  Inputs=|++
  Transpose : Math  Operator=transpose
  F_ind+F_flap : Outport
  wires:
  Constant4/1 -> Sum1/1
  Product1/1 -> Product2/1
  Sum1/1 -> Product1/1
  Constant5/1 -> Sum1/2
  psi/1 -> Mux/3
  Product2/1 -> Product3/1
  Rotation Angles to Direction Cosine Matrix/1 -> Product1/2, Transpose/1
  theta/1 -> Mux/2
  Mux/1 -> Rotation Angles to Direction Cosine Matrix/1
  Transpose/1 -> Product2/2
  phi/1 -> Mux/1
  dot_r/1 -> Product3/2
  Product3/1 -> Product/2
  Product/1 -> F_ind+F_flap/1
  T/1 -> Product/1

== matlab function MPC_1_QuadrotorModel/MATLAB Function1 ==
  data: t input; x_ref_traj output size=[N 12]; dt input; g input
function x_ref_traj = trajectory_generator(t, dt, g)
%#codegen
% Генерация эталонной траектории на горизонт N с шагом dt начиная с времени t

% Параметры восьмерки
A = 10;    % амплитуда по x
B = 6.5;   % амплитуда по y
h = 5;     % высота
w = 0.2;   % частота

N = 10;

x_ref_traj = zeros(N, 12);  % инициализация

for k = 1:N
    tk = t + (k-1)*dt;

    x = A * sin(w * tk);
    y = B * sin(w * tk) * cos(w * tk);
    z = h;

    dx = A * w * cos(w * tk);
    dy = B * w * cos(2 * w * tk);

    psi = atan2(dy, dx);  % курс

    x_ref_traj(k, :) = [x, y, z, 0, 0, 0, 0, 0, 0, 0, 0, 0];
end
end

== matlab function MPC_1_QuadrotorModel/MATLAB Function3 ==
  data: x input; y input; z input; xd input; yd input; zd input
function draw_trajectory(x, y, z, xd, yd, zd)
    coder.extrinsic('plot3');
    plot3(x, y, z, 'r');
    grid on;
    hold on;
    plot3(xd, yd, zd, 'b--');
end

== matlab function MPC_1_QuadrotorModel/MATLAB Function ==
  data: t input; x_ref_traj output; dt input; forward_20 input; forward_10 input; up_down input; total_time input
function x_ref_traj = generate_quadcopter_route_real_time(t, dt, forward_20, forward_10, up_down, total_time)
% Генерирует эталонную траекторию [N x 12] на горизонте планирования

turn_time_ratio = 0.2;
total_turn_time = total_time * turn_time_ratio;
total_linear_time = total_time - total_turn_time;
turn_time = total_turn_time / 4;
N = 10;
segments = [
    forward_20, 0, 0, 0;
    0, 0, up_down, 0;
    0, 0, 0, -pi/2;
    forward_10, 0, 0, 0;
    0, 0, -up_down, 0;
    0, 0, 0, -pi/2;
    forward_20, 0, 0, 0;
    0, 0, up_down, 0;
    0, 0, 0, -pi/2;
    forward_10, 0, 0, 0;
    0, 0, -up_down, 0;
    0, 0, 0, -pi/2;
];

segment_lengths = vecnorm(segments(:, 1:3), 2, 2);
total_path_length = sum(segment_lengths);
segment_times = zeros(size(segments, 1), 1);

for i = 1:size(segments, 1)
    if segments(i, 4) == 0
        segment_times(i) = segment_lengths(i) / total_path_length * total_linear_time;
    else
        segment_times(i) = turn_time;
    end
end

% Инициализация
current_x = 0;
current_y = 0;
current_z = 0;
current_psi = 0;
accumulated_time = 0;

% Выходная траектория
x_ref_traj = zeros(N, 12);

for k = 1:N
    tk = t + (k-1)*dt;

    % Снова инициализация для поиска нужного сегмента
    current_x = 0; current_y = 0; current_z = 0; current_psi = 0;
    accumulated_time = 0;

    for s = 1:size(segments, 1)
        dt_seg = segment_times(s);
        if tk <= accumulated_time + dt_seg || s == size(segments, 1)
            segment_progress = (tk - accumulated_time) / dt_seg;
            segment_progress = max(0, min(1, segment_progress));

            dx = segments(s, 1) * segment_progress;
            dy = segments(s, 2) * segment_progress;
            dz = segments(s, 3) * segment_progress;
            dpsi = segments(s, 4) * segment_progress;

            if dx ~= 0 || dy ~= 0
                R = [cos(current_psi), -sin(current_psi);
                     sin(current_psi),  cos(current_psi)];
                xy = R * [dx; dy];
            else
                xy = [0; 0];
            end

            x = current_x + xy(1);
            y = current_y + xy(2);
            z = current_z + dz;
            psi = current_psi + dpsi;

            x_ref_traj(k, :) = [x, y, z, 0, 0, 0, 0, 0, psi, 0, 0, 0];
            break;
        end

        % Продвигаемся по завершённым сегментам
        dx = segments(s, 1);
        dy = segments(s, 2);
        dz = segments(s, 3);
        dpsi = segments(s, 4);

        if dx ~= 0 || dy ~= 0
            R = [cos(current_psi), -sin(current_psi);
                 sin(current_psi),  cos(current_psi)];
            xy = R * [dx; dy];
        else
            xy = [0; 0];
        end

        current_x = current_x + xy(1);
        current_y = current_y + xy(2);
        current_z = current_z + dz;
        current_psi = current_psi + dpsi;
        accumulated_time = accumulated_time + dt_seg;
    end
end
end

== matlab function MPC_1_QuadrotorModel/MATLAB Function4 ==
  data: x0 input size=[12 1]; u_opt output size=4; x_ref_traj input size=[N 12]; u_ref_traj input size=[N 4]; Q input size=[12 12]; R input size=[4 4]; Ix input; Iy input; Iz input; m input; g input; U_prev input; U_all output
function [u_opt, U_all] = NMPC_Quadcopter(x0, x_ref_traj, u_ref_traj, Q, R, Ix, Iy, Iz, m, g, U_prev)
% Убрано жесткое задание Q и R из кода (используем входные параметры)
% Q = diag([1e4,1e4,1e4,  % Позиция
%           1e2,1e2,1e2,  % Скорость
%           1e4,1e4,1e4,  % Углы
%           1e2,1e2,1e2]);% Угловые скорости
% 
% R = diag([0.1, 0.01, 0.01, 0.01]); % Больший вес для тяги
%% Инициализация параметров NMPC
% Хорошие веса
% Q = diag([4e2,4e2,4e2,     1e1, 1e1, 1e1,    2e2, 2e2, 1,    1, 1, 1]);
% R = diag([20, 8, 8, 8]);
% Q = diag([3e1,3e1,5e2,     3e0, 3e0, 1e0,    1e0, 1e0, 0,    1, 1, 1]);
% R = diag([2, 0.5, 0.5, 0.5]);
Q = diag([4e2,4e2,4e2,     1e1, 1e1, 1e1,    2e2, 2e2, 0,    1, 1, 1]);
R = diag([20, 8, 8, 8]);

N = 10;                         % Увеличенный горизонт прогноза
params = struct();
params.N = N;                    
params.dt = 0.05;              % Уменьшенный шаг дискретизации
params.alpha = [0.5; 0.01; 0.01; 0.01]/5; % Обновленные коэффициенты
params.momentum = 0.95;          % Добавлен момент инерции для оптимизации
params.max_iters = 5;         % Увеличенное число итераций

% Физические параметры
params.m = m;
params.g = g;
params.Ix = Ix;
params.Iy = Iy;
params.Iz = Iz;
params.S = diag([1e4, 0, 0, 0])*0;

% Обновленные ограничения управления
params.umin = [0.1; -0.2; -0.2; -5]; % Более реалистичные пределы
params.umax = [16; 0.2; 0.2; 5];

% Инициализация
dt = params.dt;
alpha = params.alpha;
max_iters = params.max_iters;
umin = params.umin;
umax = params.umax;

if isempty(U_prev)
    U = u_ref; % если ничего не передали, начни с u_ref
else
    U = [U_prev(2:end,:); U_prev(end,:)];
end

J_min = Inf;
u_opt = U(1, :)';
velocity = zeros(size(U));      % Для момента
J_history = zeros(1, max_iters);
%% Улучшенный градиентный спуск с моментумом
for iter = 1:max_iters
    [J_total, grad_U] = compute_gradient(x0, U, x_ref_traj, u_ref_traj, Q, R, dt, params);
    
    % Адаптивное обновление с моментумом
    velocity = params.momentum * velocity - grad_U .* alpha';
    U = U + velocity;
    
    % Проекция с учетом новых ограничений
    U = max(min(U, umax'), umin');

    % Адаптивная регулировка шага
    if iter > 10 && J_history(size(J_history, 2)) > 0.9*J_history(size(J_history, 2)-1)
        alpha = 0.95*alpha; % Уменьшаем шаг при затухании сходимости
    end
    
    % Сохранение лучшего управления
    if J_total < J_min
        J_min = J_total;
        u_opt = U(1, :)';
    end
    J_history(iter) = J_total;
end
U_all = U;
end

%% Оптимизированное вычисление градиента
function [J_total, grad_U] = compute_gradient(x0, U, x_ref_traj, u_ref_traj, Q, R, dt, params)
N = params.N;
du = [0.01; 0.0050; 0.0005; 0.0005]/5; % Уменьшенные шаги возмущения
grad_U = zeros(size(U));
J_total = simulate_full_cost(x0, U, x_ref_traj, u_ref_traj, Q, R, dt, params);

parfor k = 1:N % Параллельные вычисления
    for j = 1:4
        U_pert = U;
        U_pert(k,j) = U_pert(k,j) + du(j);
        
        J_pert = simulate_full_cost(x0, U_pert, x_ref_traj, u_ref_traj, Q, R, dt, params);
        grad_U(k,j) = (J_pert - J_total)/du(j);
    end
end
end

function cost = simulate_full_cost(x0, U, x_ref_traj, u_ref_traj, Q, R, dt, params)
cost = 0;
x = x0;
N = params.N;
S = params.S;
phi_limit = pi/5;
theta_limit = pi/5;
soft_weight = 1e7; % Вес мягких ограничений

for k = 1:N
    u_k = U(k, :)';
    x_ref_k = x_ref_traj(k, :)';
    u_ref_k = u_ref_traj(k, :)';
    
    % Основной штраф
    cost = cost + (x - x_ref_k)' * Q * (x - x_ref_k) + ...
                  (u_k - u_ref_k)' * R * (u_k - u_ref_k);
    
    % Добавим soft constraint на углы
    phi = x(7); theta = x(8);
    if abs(phi) > phi_limit
        cost = cost + soft_weight * (abs(phi) - phi_limit)^2;
    end
    if abs(theta) > theta_limit
        cost = cost + soft_weight * (abs(theta) - theta_limit)^2;
    end
    if k>1
        delta_u = u_k - U(k-1, :)';
        cost = cost + delta_u' * S * delta_u;
    end
    % Следующее состояние
    x = dynamics_discrete_2(x, u_k, dt);
end
end

%% Непрерывная динамика квадрокоптера (правые части ОДУ)
function dxdt = dynamics_continuous(x, u, p)
% Входы:
%   x - текущее состояние (12x1)
%   u - управление (4x1)
%   p - параметры системы
% Выход:
%   dxdt - производные состояния (12x1)

% Распаковка состояния
rx = x(1); ry = x(2); rz = x(3);
vx = x(4); vy = x(5); vz = x(6);
phi = x(7); theta = x(8); psi = x(9);
w_phi = x(10); w_theta = x(11); w_psi = x(12);

% Распаковка управления
T = u(1); 
tau_phi = u(2); 
tau_theta = u(3); 
tau_psi = u(4);

% Параметры системы
m = p.m; 
g = p.g;
Ix = p.Ix; Iy = p.Iy; Iz = p.Iz;

% 1. Производные угловых скоростей
dw_phi = (tau_phi + (Iy - Iz)*w_theta*w_psi)/Ix;
dw_theta = (tau_theta + (Iz - Ix)*w_phi*w_psi)/Iy;
dw_psi = (tau_psi + (Ix - Iy)*w_phi*w_theta)/Iz;

% 2. Производные углов Эйлера
dphi = w_phi + tan(theta)*(w_theta*sin(phi) + w_psi*cos(phi));
dtheta = w_theta*cos(phi) - w_psi*sin(phi);
dpsi = (sin(phi)/cos(theta))*w_theta + (cos(phi)/cos(theta))*w_psi;

% 3. Ускорения в глобальной системе координат
cth = cos(theta); sth = sin(theta);
cph = cos(phi); sph = sin(phi);
cps = cos(psi); sps = sin(psi);

ax = (T/m)*(cps*sth*cph + sps*sph);
ay = (T/m)*(sps*sth*cph - cps*sph);
az = (T/m)*(cth*cph) - g;

% Сборка вектора производных
dxdt = zeros(12,1);
dxdt(1:3) = [vx; vy; vz];     % Производные позиций
dxdt(4:6) = [ax; ay; az];     % Производные скоростей
dxdt(7:9) = [dphi; dtheta; dpsi]; % Производные углов
dxdt(10:12) = [dw_phi; dw_theta; dw_psi]; % Производные угловых скоростей
end

%% Дискретная динамика с использованием RK4
function x_next = dynamics_discrete(x, u, dt, p)
% Входы:
%   x - текущее состояние (12x1)
%   u - управление (4x1)
%   dt - шаг интегрирования
%   p - параметры системы
% Выход:
%   x_next - состояние после шага интегрирования

% Вычисление коэффициентов Рунге-Кутта
k1 = dynamics_continuous(x, u, p);
k2 = dynamics_continuous(x + 0.5*dt*k1, u, p);
k3 = dynamics_continuous(x + 0.5*dt*k2, u, p);
k4 = dynamics_continuous(x + dt*k3, u, p);

% Комбинирование коэффициентов
x_next = x + (dt/6)*(k1 + 2*k2 + 2*k3 + k4);

% Применение ограничений (опционально)
% x_next(7:9) = wrapToPi(x_next(7:9)); % Для углов, если нужно
end
